simulink model "PR3_P2_Bescos_Santiago"  (R2023a)
settings: Solver=VariableStepAuto  StartTime=0.0  StopTime=30  RelTol=1e-3
libraries: simulink x1
settings Model: Creator=santi  LastModifiedBy=santi

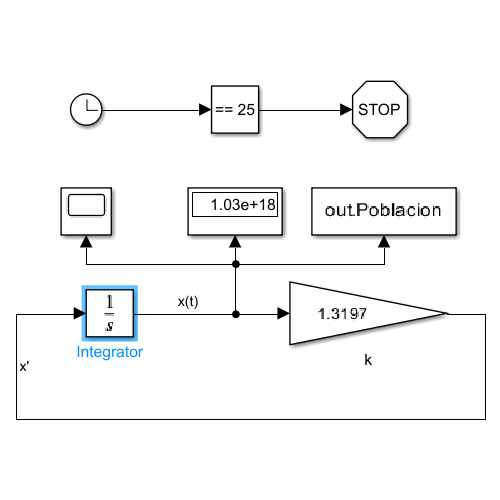
[thumbnail: Simulink's stored preview of the top-level diagram]
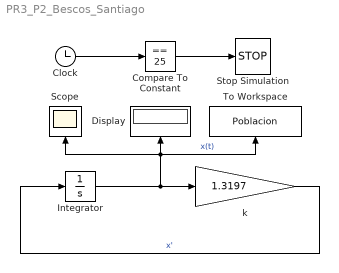
== system PR3_P2_Bescos_Santiago ==
  Clock : Clock
  Compare To Constant : simulink/Logic and Bit Operations/Compare To Constant  relop===  const=25  OutDataTypeStr=boolean
  Display : Display
  Integrator : Integrator  InitialCondition=4830
  Scope : Scope
  Stop Simulation : Stop
  To Workspace : ToWorkspace  VariableName=Poblacion  SampleTime=-1
  k : Gain  Gain=1.3197
  wires:
  Integrator/1 -> To Workspace/1, Display/1, Scope/1, k/1  "x(t)"
  Clock/1 -> Compare To Constant/1
  k/1 -> Integrator/1  "x'"
  Compare To Constant/1 -> Stop Simulation/1
